simulink model "gm_adpcm_precision_study"  (R2021a)
settings: Solver=VariableStepAuto  StartTime=0.0  StopTime=.05  RelTol=1e-3
libraries: dspstat3 x4, hdlmdlgenlib x3, dspfdesign x1, simulink x1
settings Model: Creator=jeldo  LastModifiedBy=ankursharma
settings SolverCC: AlgebraicLoopSolver=TrustRegion
settings OptimizationCC: BlockReduction=off  ConditionallyExecuteInputs=off
settings DebuggingCC: InheritedTsInSrcMsg=none  SFMachineParentedDataDiag=warning

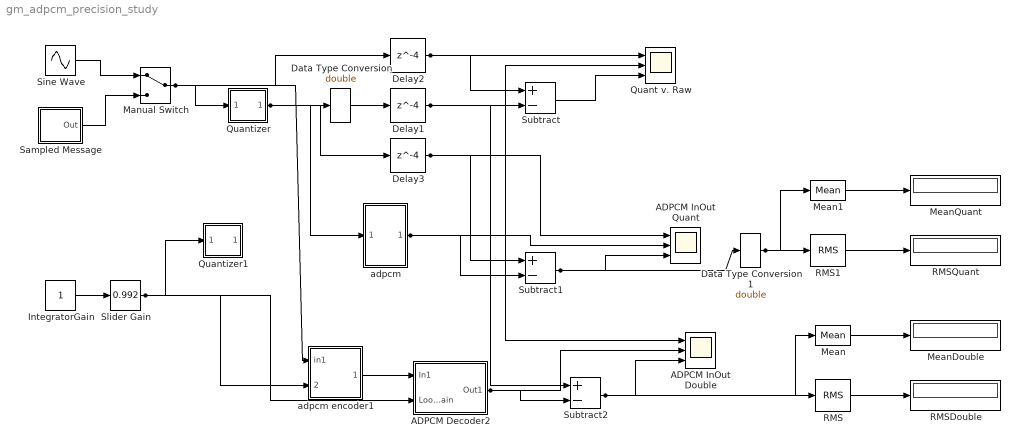
== system gm_adpcm_precision_study ==
  "  Sampled Message" : Subsystem
  ADPCM Decoder2 : Subsystem  AncestorBlock=dspwvfmcdlib/ADPCM Decoder  mask(ADPCM Decoder){StepAttn=0.5, StepGain=2, StepMax=0.5, StepMin=0.01, StepInit=0.1, AdpcmIntTau=0.99}
      mask prompts: StepAttn "Step-size attenuation"; StepGain "Step-size gain"; StepMax "Maximum step size"; StepMin "Minimum step size"; StepInit "Initial step size"; AdpcmIntTau "Integrator time constant"
      mask Display: disp('ADPCM\nDecoder')
  ADPCM InOut Double : Scope  NumInputPorts=3
  ADPCM InOut Quant : Scope  NumInputPorts=3
  Data Type Conversion : DataTypeConversion  OutDataTypeStr=double
  Data Type Conversion1 : DataTypeConversion  OutDataTypeStr=double
  Delay1 : Delay  DelayLength=4  InitialCondition=0
  Delay2 : Delay  DelayLength=4  InitialCondition=0
  Delay3 : Delay  DelayLength=4  InitialCondition=0
  IntegratorGain : Constant  SampleTime=-1
  Manual Switch : ManualSwitch
  Mean : dspstat3/Mean  run=on  InputProcessing=Columns as channels (frame based)  reset_popup=None  directionMode=Each row  dimension=1  roiEnable=off  roiType=Rectangles  roiPortion=Entire ROI  roiOutput=Individual statistics for each ROI  roiFlag=off  roundingMode=Floor  overflowMode=off  outputDataTypeStr=Inherit: Same as accumulator  outputMin=[]  outputMax=[]  outputLastDataTypeStr=Inherit: Same as accumulator
  Mean1 : dspstat3/Mean  run=on  InputProcessing=Columns as channels (frame based)  reset_popup=None  directionMode=Each row  dimension=1  roiEnable=off  roiType=Rectangles  roiPortion=Entire ROI  roiOutput=Individual statistics for each ROI  roiFlag=off  roundingMode=Floor  overflowMode=off  outputDataTypeStr=Inherit: Same as accumulator  outputMin=[]  outputMax=[]  outputLastDataTypeStr=Inherit: Same as accumulator
  MeanDouble : Display
  MeanQuant : Display
  Quant v. Raw : Scope  NumInputPorts=3
  Quantizer : Subsystem
  Quantizer1 : Subsystem
  RMS : dspstat3/RMS  run=on  directionMode=Each row  dimension=1  InputProcessing=Columns as channels (frame based)  reset_popup=None
  RMS1 : dspstat3/RMS  run=on  directionMode=Each row  dimension=1  InputProcessing=Columns as channels (frame based)  reset_popup=None
  RMSDouble : Display
  RMSQuant : Display
  Sine Wave : Sin  SineType=Sample based  Samples=1000  SampleTime=1/100000
  Slider Gain : simulink/Math Operations/Slider Gain  gain=0.992  low=.9  high=1
  Subtract : Sum  Inputs=+-
  Subtract1 : Sum  Inputs=+-
  Subtract2 : Sum  Inputs=+-
  adpcm : Subsystem
  adpcm encoder1 : Subsystem  mask(ADPCM Encoder){EncStepAttn=.5, EncStepGain=2, EncStepMax=0.5, EncStepMin=0.01, EncStepInit=0.1, EncIntTau=0.99}
      mask prompts: EncStepAttn "Step-size attenuation"; EncStepGain "Step-size gain"; EncStepMax "Maximum step size"; EncStepMin "Minimum step size"; EncStepInit "Initial step size"; EncIntTau "Integrator time constant"
      mask Display: disp('ADPCM\nEncoder')
  wires:
  adpcm/1(Out1) -> Subtract1/2, ADPCM InOut Quant/2
  Data Type Conversion1/1 -> RMS1/1, Mean1/1
  Subtract2/1 -> RMS/1, Mean/1, ADPCM InOut Double/3
  Mean1/1 -> MeanQuant/1
  RMS1/1 -> RMSQuant/1
  RMS/1 -> RMSDouble/1
  Mean/1 -> MeanDouble/1
  Delay3/1 -> ADPCM InOut Quant/1, Subtract1/1
  Delay2/1 -> Quant v. Raw/1, Subtract/1
  Quantizer/1(Out1) -> Delay3/1, adpcm/1(in1), Data Type Conversion/1
  Manual Switch/1 -> Quantizer/1(In1), adpcm encoder1/1(in1), Delay2/1
  "  Sampled Message"/1(Out) -> Manual Switch/2
  Sine Wave/1 -> Manual Switch/1
  adpcm encoder1/1(out1) -> ADPCM Decoder2/1(In1)
  ADPCM Decoder2/1(Out1) -> Subtract2/2, ADPCM InOut Double/2
  Slider Gain/1 -> adpcm encoder1/2(LoopGain), ADPCM Decoder2/2(LoopGain), Quantizer1/1(In1)
  IntegratorGain/1 -> Slider Gain/1
  Subtract1/1 -> Data Type Conversion1/1, ADPCM InOut Quant/3
  Subtract/1 -> Quant v. Raw/3
  Delay1/1 -> Subtract/2, Quant v. Raw/2, ADPCM InOut Double/1, Subtract2/1
  Data Type Conversion/1 -> Delay1/1

== system gm_adpcm_precision_study/  Sampled Message ==
  Constant : Constant  SampleTime=-1
  Gain : Gain  Gain=0.8  SaturateOnIntegerOverflow=on  OutDataTypeStr=Inherit: Same as input  ParamDataTypeStr=Inherit: Same as input
  Lowpass Filter : dspfdesign/Lowpass Filter  FilterType=FIR  DesignForMinimumOrder=on  FilterOrder=50  PassbandFrequency=250  StopbandFrequency=1000  PassbandRipple=0.2  StopbandAttenuation=40  InheritSampleRate=off  SampleRate=100000  SimulateUsing=Code generation  roundingMode=Floor  coeffsDataTypeStr=fixdt(1,16)
  Pulse Generator : DiscretePulseGenerator  Amplitude=2  Period=2000  PulseWidth=1000  SampleTime=1/100000
  Subtract : Sum  Inputs=+-
  Out : Outport
  wires:
  Constant/1 -> Subtract/2
  Subtract/1 -> Lowpass Filter/1
  Pulse Generator/1 -> Subtract/1
  Lowpass Filter/1 -> Gain/1
  Gain/1 -> Out/1

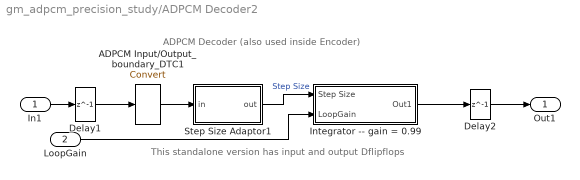
== system gm_adpcm_precision_study/ADPCM Decoder2 ==
  note: ADPCM Decoder (also used inside Encoder)
  note: This standalone version has input and output Dflipflops
  In1 : Inport
  LoopGain : Inport  Port=2
  ADPCM Input/Output_boundary_DTC1 : DataTypeConversion  SaturateOnIntegerOverflow=on  RndMeth=Zero
  Delay1 : Delay  DelayLength=1  InitialCondition=0
  Delay2 : Delay  DelayLength=1  InitialCondition=0  InputProcessing=Columns as channels (frame based)
  "Integrator -- gain = 0.99" : Subsystem
  Step Size Adaptor1 : Subsystem  mask(Step-size adaptation){Dec=StepAttn, Inc=StepGain, MaxStep=StepMax, MinStep=StepMin, InitStep=StepInit}
      mask prompts: Dec "Step-size attenuation factor:"; Inc "Step-size gain factor:"; MaxStep "Maximum step size:"; MinStep "Minimum step size:"; InitStep "Initial step size:"
      mask help: Step-size logic
      mask Display: disp('Step Size\nAdaptation')
  Out1 : Outport
  wires:
  LoopGain/1 -> "Integrator -- gain = 0.99"/2(LoopGain)
  ADPCM Input/Output_boundary_DTC1/1 -> Step Size Adaptor1/1(in)
  Delay2/1 -> Out1/1
  Delay1/1 -> ADPCM Input/Output_boundary_DTC1/1
  "Integrator -- gain = 0.99"/1(Out1) -> Delay2/1
  Step Size Adaptor1/1(out) -> "Integrator -- gain = 0.99"/1(Step Size)  "Step Size"
  In1/1 -> Delay1/1

== system gm_adpcm_precision_study/Quantizer ==
  In1 : Inport
  A/D Converter1 : ZeroOrderHold  Commented=through  SampleTime=1/10000
  ADPCM Encoder1_boundary_DTC : DataTypeConversion  OutDataTypeStr=fixdt(1,16,12)  RndMeth=Round  SaturateOnIntegerOverflow=on
  Out1 : Outport
  wires:
  ADPCM Encoder1_boundary_DTC/1 -> Out1/1
  In1/1 -> A/D Converter1/1
  A/D Converter1/1 -> ADPCM Encoder1_boundary_DTC/1

== system gm_adpcm_precision_study/Quantizer1 ==
  In1 : Inport
  A/D Converter1 : ZeroOrderHold  Commented=through  SampleTime=1/10000
  ADPCM Encoder1_boundary_DTC : DataTypeConversion  OutDataTypeStr=fixdt(1,8,4)  RndMeth=Round  SaturateOnIntegerOverflow=on
  Out1 : Outport
  wires:
  ADPCM Encoder1_boundary_DTC/1 -> Out1/1
  In1/1 -> A/D Converter1/1
  A/D Converter1/1 -> ADPCM Encoder1_boundary_DTC/1

== system gm_adpcm_precision_study/adpcm ==
  in1 : Inport  OutDataTypeStr=fixdt(1, 16, 12)  PortDimensions=1  SampleTime=1e-05
  ADPCM Decoder1 : Subsystem  mask(ADPCM Decoder){StepAttn=double(0.5), StepGain=double(2), StepMax=double(0.5), StepMin=double(0.01), StepInit=double(0.1), AdpcmIntTau=double(0.99)}
      mask prompts: StepAttn "Step-size attenuation"; StepGain "Step-size gain"; StepMax "Maximum step size"; StepMin "Minimum step size"; StepInit "Initial step size"; AdpcmIntTau "Integrator time constant"
      mask Display: disp('ADPCM\nDecoder')
  adpcm encoder2 : Subsystem  mask(ADPCM Encoder){EncStepAttn=double(0.5), EncStepGain=double(2), EncStepMax=double(0.5), EncStepMin=double(0.01), EncStepInit=double(0.1), EncIntTau=double(0.99)}
      mask prompts: EncStepAttn "Step-size attenuation"; EncStepGain "Step-size gain"; EncStepMax "Maximum step size"; EncStepMin "Minimum step size"; EncStepInit "Initial step size"; EncIntTau "Integrator time constant"
      mask Display: disp('ADPCM\nEncoder')
  Out1 : Outport  SampleTime=1e-05
  wires:
  in1/1 -> adpcm encoder2/1(in1)
  ADPCM Decoder1/1(Out1) -> Out1/1
  adpcm encoder2/1(out1) -> ADPCM Decoder1/1(In1)

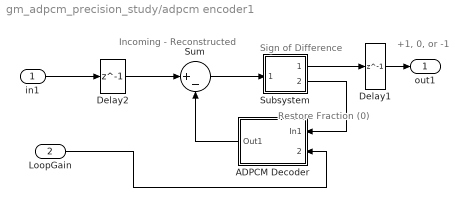
== system gm_adpcm_precision_study/adpcm encoder1 ==
  note: +1, 0, or -1
  note: Restore Fraction (0)
  note: Sign of Difference
  note: Incoming - Reconstructed
  in1 : Inport
  LoopGain : Inport  Port=2
  ADPCM Decoder : Subsystem  AncestorBlock=dspwvfmcdlib/ADPCM Decoder  mask(ADPCM Decoder){StepAttn=EncStepAttn, StepGain=EncStepGain, StepMax=EncStepMax, StepMin=EncStepMin, StepInit=EncStepInit, AdpcmIntTau=EncIntTau}
      mask prompts: StepAttn "Step-size attenuation"; StepGain "Step-size gain"; StepMax "Maximum step size"; StepMin "Minimum step size"; StepInit "Initial step size"; AdpcmIntTau "Integrator time constant"
      mask Display: disp('ADPCM\nDecoder')
  Delay1 : Delay  DelayLength=1  InitialCondition=0
  Delay2 : Delay  DelayLength=1  InitialCondition=0
  Subsystem : Subsystem
  Sum : Sum  Inputs=|+-  InputSameDT=on  SaturateOnIntegerOverflow=on  OutDataTypeStr=Inherit: Same as first input
  out1 : Outport
  wires:
  LoopGain/1 -> ADPCM Decoder/2(LoopGain)
  Delay1/1 -> out1/1
  Delay2/1 -> Sum/1
  Subsystem/2(Out2) -> ADPCM Decoder/1(In1)
  Subsystem/1(Out1) -> Delay1/1
  in1/1 -> Delay2/1
  Sum/1 -> Subsystem/1(In1)
  ADPCM Decoder/1(Out1) -> Sum/2

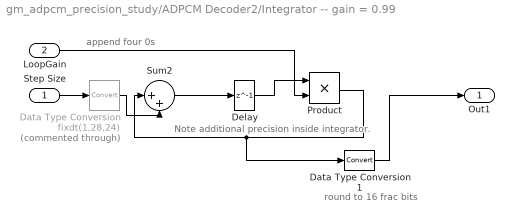
== system gm_adpcm_precision_study/ADPCM Decoder2/Integrator -- gain = 0.99 ==
  note: Note additional precision inside integrator.
  note: append four 0s
  note: round to 16 frac bits
  Step Size : Inport
  LoopGain : Inport  Port=2
  Data Type Conversion : DataTypeConversion  Commented=through  OutDataTypeStr=fixdt(1,28,24)  RndMeth=Nearest
  Data Type Conversion1 : DataTypeConversion  RndMeth=Nearest
  Delay : Delay  DelayLength=1  InitialCondition=0  InputProcessing=Columns as channels (frame based)
  Product : Product  OutDataTypeStr=Inherit: Same as first input
  Sum2 : Sum  Inputs=|++  InputSameDT=on  SaturateOnIntegerOverflow=on  OutDataTypeStr=Inherit: Same as first input
  Out1 : Outport
  wires:
  LoopGain/1 -> Product/2
  Data Type Conversion1/1 -> Out1/1
  Delay/1 -> Product/1
  Product/1 -> Data Type Conversion1/1, Sum2/1
  Step Size/1 -> Data Type Conversion/1
  Data Type Conversion/1 -> Sum2/2
  Sum2/1 -> Delay/1

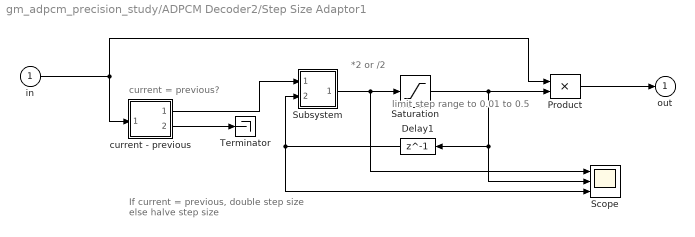
== system gm_adpcm_precision_study/ADPCM Decoder2/Step Size Adaptor1 ==
  note: limit step range
      | to 0.01 to 0.5
  note: *2 or /2
  note: current = previous?
  note: If current = previous, double step size
      | else halve step size
  in : Inport
  Delay1 : Delay  DelayLength=1  InitialCondition=13/128  InputProcessing=Columns as channels (frame based)
  Product : Product  InputSameDT=on  RndMeth=Convergent  SaturateOnIntegerOverflow=on  OutDataTypeStr=Inherit: Same as first input
  Saturation : Saturate  UpperLimit=MaxStep  LowerLimit=328/65536
  Scope : Scope  NumInputPorts=3
  Subsystem : Subsystem
  Terminator : Terminator
  current - previous : Subsystem
  out : Outport  InitialOutput=0
  wires:
  current - previous/2(Out2) -> Terminator/1
  Product/1 -> out/1
  in/1 -> current - previous/1(In1), Product/1
  current - previous/1(Out1) -> Subsystem/1(In1)
  Subsystem/1(Out1) -> Saturation/1, Scope/1
  Delay1/1 -> Subsystem/2(In2), Scope/3
  Saturation/1 -> Delay1/1, Scope/2, Product/2

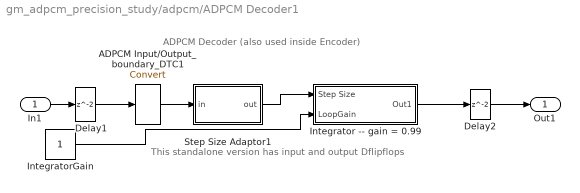
== system gm_adpcm_precision_study/adpcm/ADPCM Decoder1 ==
  note: ADPCM Decoder (also used inside Encoder)
  note: This standalone version has input and output Dflipflops
  In1 : Inport  OutDataTypeStr=fixdt(1, 2, 0)  PortDimensions=1  SampleTime=1e-05
  ADPCM Input/Output_boundary_DTC1 : DataTypeConversion  SaturateOnIntegerOverflow=on  RndMeth=Zero
  Delay1 : Delay  InitialCondition=0
  Delay2 : Delay  InitialCondition=0  InputProcessing=Columns as channels (frame based)
  "Integrator -- gain = 0.99" : Subsystem
  IntegratorGain : Constant  OutDataTypeStr=fixdt(1,20,16)  SampleTime=-1
  Step Size Adaptor1 : Subsystem  mask(Step-size adaptation){Dec=double(0.5), Inc=double(2), MaxStep=double(0.5), MinStep=double(0.01), InitStep=double(0.1)}
      mask prompts: Dec "Step-size attenuation factor:"; Inc "Step-size gain factor:"; MaxStep "Maximum step size:"; MinStep "Minimum step size:"; InitStep "Initial step size:"
      mask help: Step-size logic
      mask Display: disp('Step Size\nAdaptation')
  Out1 : Outport  SampleTime=1e-05
  wires:
  ADPCM Input/Output_boundary_DTC1/1 -> Step Size Adaptor1/1(in)
  Delay1/1 -> ADPCM Input/Output_boundary_DTC1/1
  Delay2/1 -> Out1/1
  "Integrator -- gain = 0.99"/1(Out1) -> Delay2/1
  IntegratorGain/1 -> "Integrator -- gain = 0.99"/2(LoopGain)
  Step Size Adaptor1/1(out) -> "Integrator -- gain = 0.99"/1(Step Size)
  In1/1 -> Delay1/1

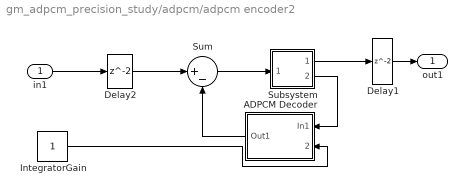
== system gm_adpcm_precision_study/adpcm/adpcm encoder2 ==
  in1 : Inport  OutDataTypeStr=fixdt(1, 16, 12)  PortDimensions=1  SampleTime=1e-05
  ADPCM Decoder : Subsystem  mask(ADPCM Decoder){StepAttn=double(0.5), StepGain=double(2), StepMax=double(0.5), StepMin=double(0.01), StepInit=double(0.1), AdpcmIntTau=double(0.99)}
      mask prompts: StepAttn "Step-size attenuation"; StepGain "Step-size gain"; StepMax "Maximum step size"; StepMin "Minimum step size"; StepInit "Initial step size"; AdpcmIntTau "Integrator time constant"
      mask Display: disp('ADPCM\nDecoder')
  Delay1 : Delay  InitialCondition=0
  Delay2 : Delay  InitialCondition=0
  IntegratorGain : Constant  OutDataTypeStr=fixdt(1,20,16)  SampleTime=-1
  Subsystem : Subsystem
  Sum : Sum  Inputs=|+-  InputSameDT=on  SaturateOnIntegerOverflow=on  OutDataTypeStr=Inherit: Same as first input
  out1 : Outport  SampleTime=1e-05
  wires:
  Delay1/1 -> out1/1
  Delay2/1 -> Sum/1
  IntegratorGain/1 -> ADPCM Decoder/2(LoopGain)
  Subsystem/1(Out1) -> Delay1/1
  in1/1 -> Delay2/1
  Sum/1 -> Subsystem/1(In1)
  ADPCM Decoder/1(Out1) -> Sum/2
  Subsystem/2(Out2) -> ADPCM Decoder/1(In1)

== system gm_adpcm_precision_study/adpcm encoder1/ADPCM Decoder ==
  In1 : Inport
  LoopGain : Inport  Port=2
  "Integrator -- gain = 0.99" : Subsystem
  Step Size Adaptor1 : Subsystem  mask(Step-size adaptation){Dec=StepAttn, Inc=StepGain, MaxStep=StepMax, MinStep=StepMin, InitStep=StepInit}
      mask prompts: Dec "Step-size attenuation factor:"; Inc "Step-size gain factor:"; MaxStep "Maximum step size:"; MinStep "Minimum step size:"; InitStep "Initial step size:"
      mask help: Step-size logic
      mask Display: disp('Step Size\nAdaptation')
  Out1 : Outport
  wires:
  LoopGain/1 -> "Integrator -- gain = 0.99"/2(LoopGain)
  "Integrator -- gain = 0.99"/1(Out1) -> Out1/1
  Step Size Adaptor1/1(out) -> "Integrator -- gain = 0.99"/1(StepSize)  "Step Size"
  In1/1 -> Step Size Adaptor1/1(in)

== system gm_adpcm_precision_study/adpcm encoder1/Subsystem ==
  note: sign extraction
  In1 : Inport
  Data Type Conversion : DataTypeConversion  OutDataTypeStr=double  RndMeth=Nearest  SaturateOnIntegerOverflow=on  LockScale=on
  Data Type Conversion1 : DataTypeConversion  OutDataTypeStr=fixdt(1,2,0)  RndMeth=Nearest  SaturateOnIntegerOverflow=on  LockScale=on
  Sign : Signum  ZeroCross=off
  Out1 : Outport
  Out2 : Outport  Port=2
  wires:
  Data Type Conversion1/1 -> Out1/1
  In1/1 -> Sign/1
  Sign/1 -> Data Type Conversion/1, Data Type Conversion1/1
  Data Type Conversion/1 -> Out2/1

== system gm_adpcm_precision_study/ADPCM Decoder2/Step Size Adaptor1/Subsystem ==
  In1 : Inport
  In2 : Inport  Port=2
  Constant1 : Constant  Value=2  OutDataTypeStr=Inherit: Inherit via back propagation  SampleTime=-1
  Constant3 : Constant  Value=0.5  OutDataTypeStr=Inherit: Inherit via back propagation  SampleTime=-1
  Product1 : Product  InputSameDT=on  RndMeth=Zero  SaturateOnIntegerOverflow=on  OutDataTypeStr=Inherit: Same as first input
  Switch : Switch  Threshold=1  SaturateOnIntegerOverflow=on  InputSameDT=on
  Out1 : Outport
  wires:
  In1/1 -> Switch/2
  Constant1/1 -> Switch/1
  Constant3/1 -> Switch/3
  Product1/1 -> Out1/1
  Switch/1 -> Product1/1
  In2/1 -> Product1/2

== system gm_adpcm_precision_study/ADPCM Decoder2/Step Size Adaptor1/current - previous ==
  In1 : Inport
  Constant5 : Constant  Value=0  OutDataTypeStr=double  SampleTime=1/100000
  Delay : Delay  DelayLength=1  InitialCondition=0  InputProcessing=Columns as channels (frame based)
  Relational Operator5 : RelationalOperator  Operator===  OutDataTypeStr=boolean  RndMeth=Nearest  InputSameDT=on
  Sum1 : Sum  Inputs=+-|  InputSameDT=on  SaturateOnIntegerOverflow=on  OutDataTypeStr=Inherit: Same as first input
  Out1 : Outport
  Out2 : Outport  Port=2
  wires:
  Relational Operator5/1 -> Out1/1
  In1/1 -> Sum1/1, Delay/1
  Sum1/1 -> Relational Operator5/1, Out2/1
  Delay/1 -> Sum1/2
  Constant5/1 -> Relational Operator5/2

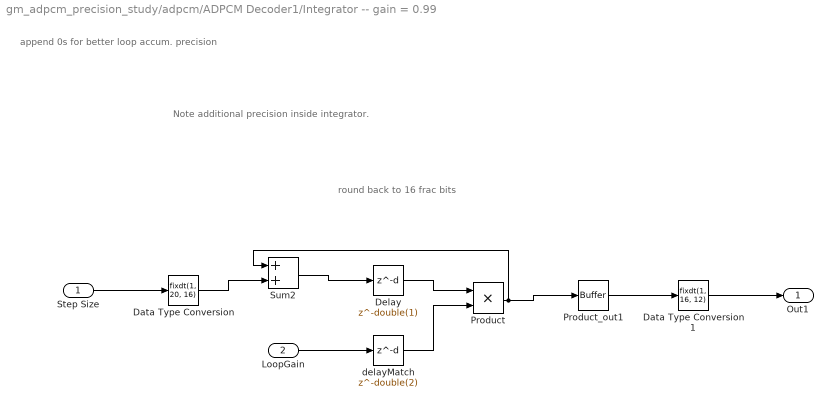
== system gm_adpcm_precision_study/adpcm/ADPCM Decoder1/Integrator -- gain = 0.99 ==
  note: Note additional precision inside integrator.
  note: append 0s for better loop accum. precision
  note: round back to 16 frac bits
  Step Size : Inport  OutDataTypeStr=fixdt(1, 16, 12)  PortDimensions=1  SampleTime=1e-05
  LoopGain : Inport  Port=2  OutDataTypeStr=fixdt(1, 20, 16)  PortDimensions=1  SampleTime=1e-05
  Data Type Conversion : DataTypeConversion  OutDataTypeStr=fixdt(1, 20, 16)  RndMeth=Nearest  SampleTime=1e-05
  Data Type Conversion1 : DataTypeConversion  OutDataTypeStr=fixdt(1, 16, 12)  RndMeth=Nearest  SampleTime=1e-05
  Delay : Delay  DelayLength=double(1)  InitialCondition=0  SampleTime=1e-05
  Product : Product  Inputs=**  OutDataTypeStr=fixdt(1, 20, 16)  RndMeth=Nearest  SampleTime=1e-05
  Product_out1 : hdlmdlgenlib/Buffer
      settings: SourceProductBaseCode=SL
  Sum2 : Sum  AccumDataTypeStr=fixdt(1, 20, 16)  OutDataTypeStr=fixdt(1, 20, 16)  SaturateOnIntegerOverflow=on  SampleTime=1e-05
  delayMatch : Delay  DelayLength=double(2)  InitialCondition=0  SampleTime=1e-05
  Out1 : Outport  SampleTime=1e-05
  wires:
  delayMatch/1 -> Product/2
  Data Type Conversion/1 -> Sum2/2
  Data Type Conversion1/1 -> Out1/1
  Product_out1/1 -> Data Type Conversion1/1
  Step Size/1 -> Data Type Conversion/1
  LoopGain/1 -> delayMatch/1
  Sum2/1 -> Delay/1
  Delay/1 -> Product/1
  Product/1 -> Product_out1/1, Sum2/1

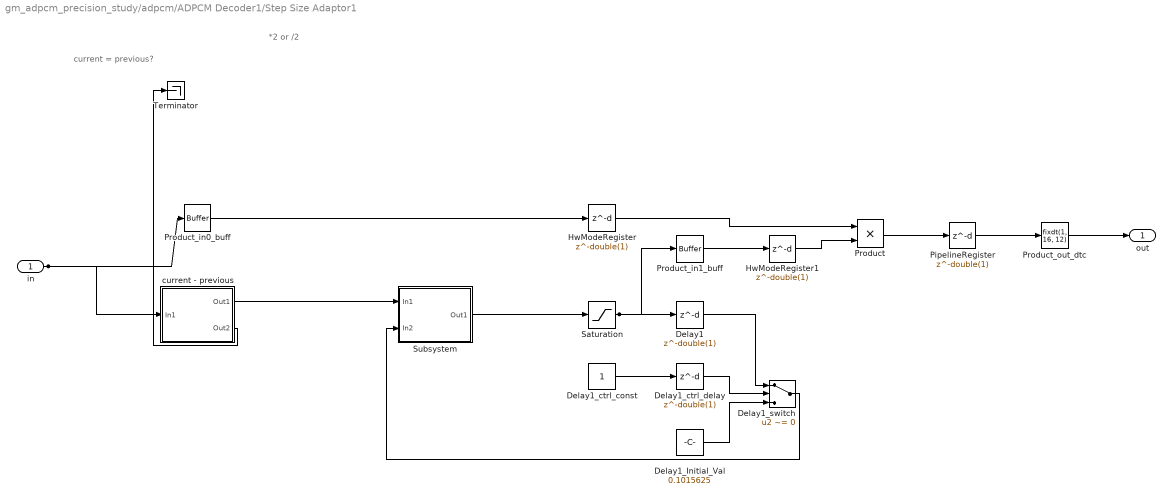
== system gm_adpcm_precision_study/adpcm/ADPCM Decoder1/Step Size Adaptor1 ==
  note: *2 or /2
  note: current = previous?
  in : Inport  OutDataTypeStr=fixdt(1, 16, 12)  PortDimensions=1  SampleTime=1e-05
  Delay1 : Delay  DelayLength=double(1)  InitialCondition=0  SampleTime=1e-05
  Delay1_Initial_Val : Constant  Value=0.1015625  OutDataTypeStr=fixdt(1, 16, 12)  SampleTime=1e-05
  Delay1_ctrl_const : Constant  OutDataTypeStr=boolean  SampleTime=1e-05
  Delay1_ctrl_delay : Delay  DelayLength=double(1)  InitialCondition=0  SampleTime=1e-05
  Delay1_switch : Switch  Criteria=u2 ~= 0  Threshold=double(0)  OutDataTypeStr=fixdt(1, 16, 12)  SampleTime=1e-05
  HwModeRegister : Delay  DelayLength=double(1)  InitialCondition=0  SampleTime=1e-05
  HwModeRegister1 : Delay  DelayLength=double(1)  InitialCondition=0  SampleTime=1e-05
  PipelineRegister : Delay  DelayLength=double(1)  InitialCondition=0  SampleTime=1e-05
  Product : Product  Inputs=**  OutDataTypeStr=fixdt(1, 32, 24)  SampleTime=1e-05
  Product_in0_buff : hdlmdlgenlib/Buffer
      settings: SourceProductBaseCode=SL
  Product_in1_buff : hdlmdlgenlib/Buffer
      settings: SourceProductBaseCode=SL
  Product_out_dtc : DataTypeConversion  OutDataTypeStr=fixdt(1, 16, 12)  RndMeth=Convergent  SampleTime=1e-05  SaturateOnIntegerOverflow=on
  Saturation : Saturate  UpperLimit="fi(0,1,16,12,\"hex\",\"0800\")"  LowerLimit="fi(0,1,16,12,\"hex\",\"0015\")"  SampleTime=1e-05  OutDataTypeStr=fixdt(1, 16, 12)
  Subsystem : Subsystem
  Terminator : Terminator
  current - previous : Subsystem
  out : Outport  SampleTime=1e-05  InitialOutput=0
  wires:
  Product_out_dtc/1 -> out/1
  Saturation/1 -> Product_in1_buff/1, Delay1/1
  current - previous/1(Out1) -> Subsystem/1(In1)
  current - previous/2(Out2) -> Terminator/1
  Delay1_Initial_Val/1 -> Delay1_switch/3
  Delay1_ctrl_const/1 -> Delay1_ctrl_delay/1
  Delay1_ctrl_delay/1 -> Delay1_switch/2
  PipelineRegister/1 -> Product_out_dtc/1
  in/1 -> Product_in0_buff/1, current - previous/1(In1)
  Delay1/1 -> Delay1_switch/1
  Delay1_switch/1 -> Subsystem/2(In2)
  Subsystem/1(Out1) -> Saturation/1
  Product/1 -> PipelineRegister/1
  HwModeRegister/1 -> Product/1
  HwModeRegister1/1 -> Product/2
  Product_in0_buff/1 -> HwModeRegister/1
  Product_in1_buff/1 -> HwModeRegister1/1

== system gm_adpcm_precision_study/adpcm/adpcm encoder2/ADPCM Decoder ==
  In1 : Inport  OutDataTypeStr=fixdt(1, 16, 12)  PortDimensions=1  SampleTime=1e-05
  LoopGain : Inport  Port=2  OutDataTypeStr=fixdt(1, 20, 16)  PortDimensions=1  SampleTime=1e-05
  "Integrator -- gain = 0.99" : Subsystem
  Step Size Adaptor1 : Subsystem  mask(Step-size adaptation){Dec=double(0.5), Inc=double(2), MaxStep=double(0.5), MinStep=double(0.01), InitStep=double(0.1)}
      mask prompts: Dec "Step-size attenuation factor:"; Inc "Step-size gain factor:"; MaxStep "Maximum step size:"; MinStep "Minimum step size:"; InitStep "Initial step size:"
      mask help: Step-size logic
      mask Display: disp('Step Size\nAdaptation')
  Out1 : Outport  SampleTime=1e-05
  wires:
  In1/1 -> Step Size Adaptor1/1(in)
  LoopGain/1 -> "Integrator -- gain = 0.99"/2(LoopGain)
  "Integrator -- gain = 0.99"/1(Out1) -> Out1/1
  Step Size Adaptor1/1(out) -> "Integrator -- gain = 0.99"/1(StepSize)

== system gm_adpcm_precision_study/adpcm/adpcm encoder2/Subsystem ==
  note: sign extraction
  In1 : Inport  OutDataTypeStr=fixdt(1, 16, 12)  PortDimensions=1  SampleTime=1e-05
  Data Type Conversion : DataTypeConversion  OutDataTypeStr=fixdt(1,16,12)  RndMeth=Nearest  SaturateOnIntegerOverflow=on  LockScale=on
  Data Type Conversion1 : DataTypeConversion  OutDataTypeStr=fixdt(1,2,0)  RndMeth=Nearest  SaturateOnIntegerOverflow=on  LockScale=on
  Sign : Signum  ZeroCross=off
  Out1 : Outport  SampleTime=1e-05
  Out2 : Outport  Port=2  SampleTime=1e-05
  wires:
  In1/1 -> Sign/1
  Data Type Conversion/1 -> Out2/1
  Data Type Conversion1/1 -> Out1/1
  Sign/1 -> Data Type Conversion1/1, Data Type Conversion/1

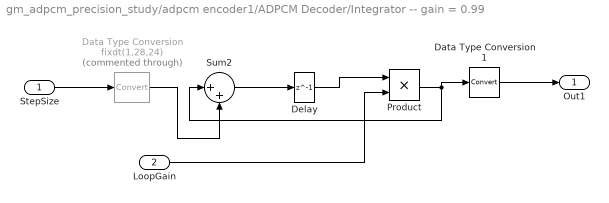
== system gm_adpcm_precision_study/adpcm encoder1/ADPCM Decoder/Integrator -- gain = 0.99 ==
  StepSize : Inport
  LoopGain : Inport  Port=2
  Data Type Conversion : DataTypeConversion  Commented=through  OutDataTypeStr=fixdt(1,28,24)  RndMeth=Nearest
  Data Type Conversion1 : DataTypeConversion  RndMeth=Convergent
  Delay : Delay  DelayLength=1  InitialCondition=0  InputProcessing=Columns as channels (frame based)
  Product : Product  RndMeth=Convergent  OutDataTypeStr=Inherit: Same as first input
  Sum2 : Sum  Inputs=|++  InputSameDT=on  SaturateOnIntegerOverflow=on  OutDataTypeStr=Inherit: Same as first input
  Out1 : Outport
  wires:
  LoopGain/1 -> Product/2
  Product/1 -> Data Type Conversion1/1, Sum2/1
  Delay/1 -> Product/1
  StepSize/1 -> Data Type Conversion/1
  Data Type Conversion/1 -> Sum2/2
  Data Type Conversion1/1 -> Out1/1
  Sum2/1 -> Delay/1

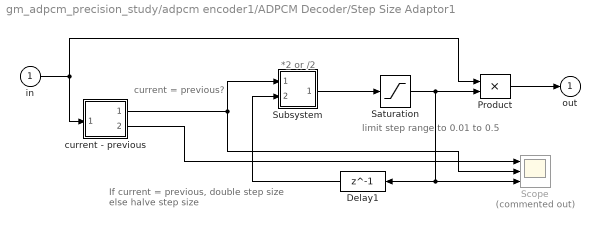
== system gm_adpcm_precision_study/adpcm encoder1/ADPCM Decoder/Step Size Adaptor1 ==
  note: limit step range
      | to 0.01 to 0.5
  note: *2 or /2
  note: current = previous?
  note: If current = previous, double step size
      | else halve step size
  in : Inport
  Delay1 : Delay  DelayLength=1  InitialCondition=13/128  InputProcessing=Columns as channels (frame based)
  Product : Product  InputSameDT=on  OutDataTypeStr=double  RndMeth=Convergent  SaturateOnIntegerOverflow=on
  Saturation : Saturate  LowerLimit=328/65536  LinearizeAsGain=off
  Scope : Scope  Commented=on  NumInputPorts=3
  Subsystem : Subsystem
  current - previous : Subsystem
  out : Outport  InitialOutput=0
  wires:
  current - previous/2(Out2) -> Scope/1
  current - previous/1(Out1) -> Subsystem/1(In1), Scope/2
  Subsystem/1(Out1) -> Saturation/1
  Delay1/1 -> Subsystem/2(In2)
  Saturation/1 -> Product/2, Delay1/1, Scope/3
  Product/1 -> out/1
  in/1 -> Product/1, current - previous/1(In1)

== system gm_adpcm_precision_study/adpcm/ADPCM Decoder1/Step Size Adaptor1/Subsystem ==
  In1 : Inport  OutDataTypeStr=boolean  PortDimensions=1  SampleTime=1e-05
  In2 : Inport  Port=2  OutDataTypeStr=fixdt(1, 16, 12)  PortDimensions=1  SampleTime=1e-05
  Constant1 : Constant  Value=2  OutDataTypeStr=fixdt(1, 16, 12)  SampleTime=1e-05
  Constant3 : Constant  Value=0.5  OutDataTypeStr=fixdt(1, 16, 12)  SampleTime=1e-05
  Product1 : Product  Inputs=**  OutDataTypeStr=fixdt(1, 16, 12)  RndMeth=Zero  SaturateOnIntegerOverflow=on  SampleTime=1e-05
  Switch : Switch  Threshold=double(1)  OutDataTypeStr=fixdt(1, 16, 12)  SampleTime=1e-05  SaturateOnIntegerOverflow=on
  Out1 : Outport  SampleTime=1e-05
  wires:
  In1/1 -> Switch/2
  In2/1 -> Product1/2
  Constant1/1 -> Switch/1
  Constant3/1 -> Switch/3
  Product1/1 -> Out1/1
  Switch/1 -> Product1/1

== system gm_adpcm_precision_study/adpcm/ADPCM Decoder1/Step Size Adaptor1/current - previous ==
  In1 : Inport  OutDataTypeStr=fixdt(1, 16, 12)  PortDimensions=1  SampleTime=1e-05
  Constant5 : Constant  Value=0  OutDataTypeStr=fixdt(1, 16, 12)  SampleTime=1e-05
  Delay : Delay  DelayLength=double(1)  InitialCondition=0  SampleTime=1e-05
  Relational Operator5 : RelationalOperator  Operator===  OutDataTypeStr=boolean  SampleTime=1e-05  RndMeth=Nearest  InputSameDT=on
  Sum1 : Sum  Inputs=+-  AccumDataTypeStr=fixdt(1, 16, 12)  OutDataTypeStr=fixdt(1, 16, 12)  SaturateOnIntegerOverflow=on  SampleTime=1e-05
  Out1 : Outport  SampleTime=1e-05
  Out2 : Outport  Port=2  SampleTime=1e-05
  wires:
  Constant5/1 -> Relational Operator5/2
  Delay/1 -> Sum1/2
  Relational Operator5/1 -> Out1/1
  Sum1/1 -> Relational Operator5/1, Out2/1
  In1/1 -> Sum1/1, Delay/1

== system gm_adpcm_precision_study/adpcm/adpcm encoder2/ADPCM Decoder/Integrator -- gain = 0.99 ==
  StepSize : Inport  OutDataTypeStr=fixdt(1, 16, 12)  PortDimensions=1  SampleTime=1e-05
  LoopGain : Inport  Port=2  OutDataTypeStr=fixdt(1, 20, 16)  PortDimensions=1  SampleTime=1e-05
  Data Type Conversion : DataTypeConversion  OutDataTypeStr=fixdt(1,20,16)  RndMeth=Nearest
  Data Type Conversion1 : DataTypeConversion  RndMeth=Convergent
  Delay : Delay  DelayLength=1  InitialCondition=0  InputProcessing=Columns as channels (frame based)
  Product : Product  RndMeth=Convergent  OutDataTypeStr=Inherit: Same as first input
  Sum2 : Sum  Inputs=|++  InputSameDT=on  SaturateOnIntegerOverflow=on  OutDataTypeStr=Inherit: Same as first input
  Out1 : Outport  SampleTime=1e-05
  wires:
  StepSize/1 -> Data Type Conversion/1
  LoopGain/1 -> Product/2
  Data Type Conversion/1 -> Sum2/2
  Data Type Conversion1/1 -> Out1/1
  Delay/1 -> Product/1
  Product/1 -> Sum2/1, Data Type Conversion1/1
  Sum2/1 -> Delay/1

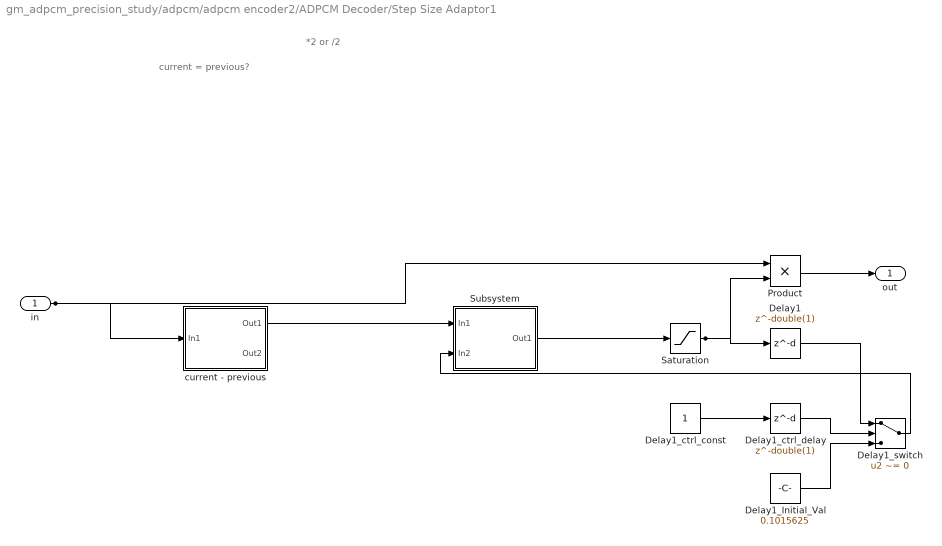
== system gm_adpcm_precision_study/adpcm/adpcm encoder2/ADPCM Decoder/Step Size Adaptor1 ==
  note: *2 or /2
  note: current = previous?
  in : Inport  OutDataTypeStr=fixdt(1, 16, 12)  PortDimensions=1  SampleTime=1e-05
  Delay1 : Delay  DelayLength=double(1)  InitialCondition=0  SampleTime=1e-05
  Delay1_Initial_Val : Constant  Value=0.1015625  OutDataTypeStr=fixdt(1, 16, 12)  SampleTime=1e-05
  Delay1_ctrl_const : Constant  OutDataTypeStr=boolean  SampleTime=1e-05
  Delay1_ctrl_delay : Delay  DelayLength=double(1)  InitialCondition=0  SampleTime=1e-05
  Delay1_switch : Switch  Criteria=u2 ~= 0  Threshold=double(0)  OutDataTypeStr=fixdt(1, 16, 12)  SampleTime=1e-05
  Product : Product  Inputs=**  OutDataTypeStr=fixdt(1, 16, 12)  RndMeth=Convergent  SaturateOnIntegerOverflow=on  SampleTime=1e-05
  Saturation : Saturate  UpperLimit="fi(0,1,16,12,\"hex\",\"0800\")"  LowerLimit="fi(0,1,16,12,\"hex\",\"0015\")"  SampleTime=1e-05  OutDataTypeStr=fixdt(1, 16, 12)
  Subsystem : Subsystem
  current - previous : Subsystem
  out : Outport  SampleTime=1e-05  InitialOutput=0
  wires:
  in/1 -> Product/1, current - previous/1(In1)
  Delay1_switch/1 -> Subsystem/2(In2)
  Product/1 -> out/1
  Saturation/1 -> Product/2, Delay1/1
  Subsystem/1(Out1) -> Saturation/1
  current - previous/1(Out1) -> Subsystem/1(In1)
  Delay1/1 -> Delay1_switch/1
  Delay1_Initial_Val/1 -> Delay1_switch/3
  Delay1_ctrl_const/1 -> Delay1_ctrl_delay/1
  Delay1_ctrl_delay/1 -> Delay1_switch/2

== system gm_adpcm_precision_study/adpcm encoder1/ADPCM Decoder/Step Size Adaptor1/Subsystem ==
  In1 : Inport
  In2 : Inport  Port=2
  Constant1 : Constant  Value=2  OutDataTypeStr=Inherit: Inherit via back propagation  SampleTime=-1
  Constant3 : Constant  Value=0.5  OutDataTypeStr=Inherit: Inherit via back propagation  SampleTime=-1
  Product1 : Product  InputSameDT=on  RndMeth=Zero  SaturateOnIntegerOverflow=on  OutDataTypeStr=Inherit: Same as first input
  Switch : Switch  Threshold=1  SaturateOnIntegerOverflow=on  InputSameDT=on
  Out1 : Outport
  wires:
  In1/1 -> Switch/2
  Constant1/1 -> Switch/1
  Constant3/1 -> Switch/3
  Product1/1 -> Out1/1
  Switch/1 -> Product1/1
  In2/1 -> Product1/2

== system gm_adpcm_precision_study/adpcm encoder1/ADPCM Decoder/Step Size Adaptor1/current - previous ==
  In1 : Inport
  Constant5 : Constant  Value=0  OutDataTypeStr=double  SampleTime=-1
  Delay : Delay  DelayLength=1  InitialCondition=0  InputProcessing=Columns as channels (frame based)
  Relational Operator5 : RelationalOperator  Operator===  OutDataTypeStr=boolean  RndMeth=Nearest  InputSameDT=on
  Sum1 : Sum  Inputs=+-|  InputSameDT=on  AccumDataTypeStr=double  SaturateOnIntegerOverflow=on  OutDataTypeStr=Inherit: Same as first input
  Out1 : Outport
  Out2 : Outport  Port=2
  wires:
  Relational Operator5/1 -> Out1/1
  In1/1 -> Sum1/1, Delay/1
  Sum1/1 -> Relational Operator5/1, Out2/1
  Delay/1 -> Sum1/2
  Constant5/1 -> Relational Operator5/2

== system gm_adpcm_precision_study/adpcm/adpcm encoder2/ADPCM Decoder/Step Size Adaptor1/Subsystem ==
  In1 : Inport  OutDataTypeStr=boolean  PortDimensions=1  SampleTime=1e-05
  In2 : Inport  Port=2  OutDataTypeStr=fixdt(1, 16, 12)  PortDimensions=1  SampleTime=1e-05
  Constant1 : Constant  Value=2  OutDataTypeStr=fixdt(1, 16, 12)  SampleTime=1e-05
  Constant3 : Constant  Value=0.5  OutDataTypeStr=fixdt(1, 16, 12)  SampleTime=1e-05
  Product1 : Product  Inputs=**  OutDataTypeStr=fixdt(1, 16, 12)  RndMeth=Zero  SaturateOnIntegerOverflow=on  SampleTime=1e-05
  Switch : Switch  Threshold=double(1)  OutDataTypeStr=fixdt(1, 16, 12)  SampleTime=1e-05  SaturateOnIntegerOverflow=on
  Out1 : Outport  SampleTime=1e-05
  wires:
  In1/1 -> Switch/2
  In2/1 -> Product1/2
  Constant1/1 -> Switch/1
  Constant3/1 -> Switch/3
  Product1/1 -> Out1/1
  Switch/1 -> Product1/1

== system gm_adpcm_precision_study/adpcm/adpcm encoder2/ADPCM Decoder/Step Size Adaptor1/current - previous ==
  In1 : Inport  OutDataTypeStr=fixdt(1, 16, 12)  PortDimensions=1  SampleTime=1e-05
  Constant5 : Constant  Value=0  OutDataTypeStr=fixdt(1, 16, 12)  SampleTime=1e-05
  Delay : Delay  DelayLength=double(1)  InitialCondition=0  SampleTime=1e-05
  Relational Operator5 : RelationalOperator  Operator===  OutDataTypeStr=boolean  SampleTime=1e-05  RndMeth=Nearest  InputSameDT=on
  Sum1 : Sum  Inputs=+-  AccumDataTypeStr=fixdt(1, 16, 12)  OutDataTypeStr=fixdt(1, 16, 12)  SaturateOnIntegerOverflow=on  SampleTime=1e-05
  Out1 : Outport  SampleTime=1e-05
  Out2 : Outport  Port=2  SampleTime=1e-05
  wires:
  In1/1 -> Sum1/1, Delay/1
  Constant5/1 -> Relational Operator5/2
  Delay/1 -> Sum1/2
  Relational Operator5/1 -> Out1/1
  Sum1/1 -> Relational Operator5/1, Out2/1
